simulink model "invPend_Linearization_op_point"  (R2020a)
settings: Solver=VariableStepAuto  StartTime=0.0  StopTime=10  RelTol=1e-3
values from neighbouring files (symbols this model uses):
  delta = 0.25    [test_inv_pendulum_linearization.m]
  g = 9.81    [test_inv_pendulum_linearization.m]
  l = 1    [test_inv_pendulum_linearization.m]
  u0 = 0    [test_inv_pendulum_linearization.m]
undefined symbols (not defined in the file or in its folder): A, B, C, D, y0
settings Model: Creator=mircea  LastModifiedBy=mircea

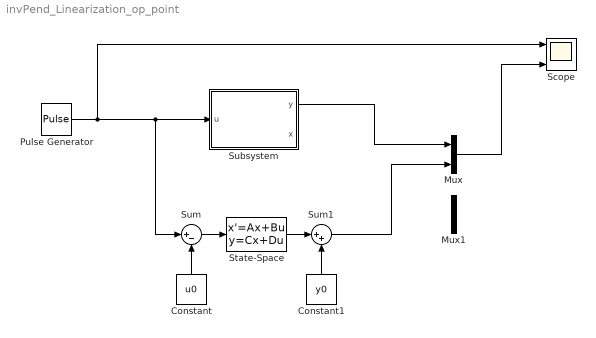
== system invPend_Linearization_op_point ==
  Constant : Constant  Value=u0
  Constant1 : Constant  Value=y0
  Mux : Mux  Inputs=2
  Mux1 : Mux  Inputs=2
  Pulse Generator : DiscretePulseGenerator  PulseType=Time based  Period=10  PulseWidth=10
  Scope : Scope  NumInputPorts=3
  State-Space : StateSpace  A=A  B=B  C=C  D=D  InitialCondition=0
  Subsystem : Subsystem
  Sum : Sum  Inputs=|+-
  Sum1 : Sum  Inputs=|++
  wires:
  Pulse Generator/1 -> Scope/1, Sum/1, Subsystem/1(u)
  Sum/1 -> State-Space/1
  State-Space/1 -> Sum1/1
  Sum1/1 -> Mux/2
  Subsystem/1(y) -> Mux/1
  Mux/1 -> Scope/3
  Constant/1 -> Sum/2
  Constant1/1 -> Sum1/2

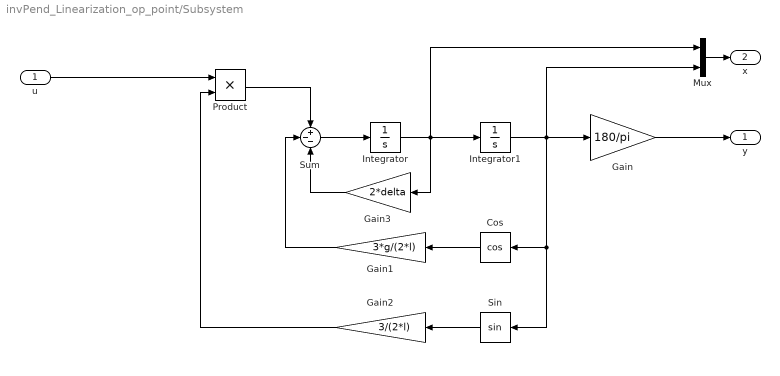
== system invPend_Linearization_op_point/Subsystem ==
  u : Inport
  Cos : Trigonometry  Operator=cos
  Gain : Gain  Gain=180/pi
  Gain1 : Gain  Gain=3*g/(2*l)
  Gain2 : Gain  Gain=3/(2*l)
  Gain3 : Gain  Gain=2*delta
  Integrator : Integrator
  Integrator1 : Integrator  InitialCondition=pi/2
  Mux : Mux  Inputs=2
  Product : Product
  Sin : Trigonometry
  Sum : Sum  Inputs=+--
  y : Outport
  x : Outport  Port=2
  wires:
  Product/1 -> Sum/1
  u/1 -> Product/1
  Integrator1/1 -> Mux/2, Sin/1, Cos/1, Gain/1
  Gain3/1 -> Sum/3
  Sum/1 -> Integrator/1
  Gain/1 -> y/1
  Sin/1 -> Gain2/1
  Cos/1 -> Gain1/1
  Integrator/1 -> Mux/1, Gain3/1, Integrator1/1
  Gain1/1 -> Sum/2
  Gain2/1 -> Product/2
  Mux/1 -> x/1
